simulink model "plant_test"  (R2018a)
settings: Solver=VariableStepAuto  StartTime=0.0  StopTime=10.0  RelTol=1e-3
settings Model: Creator=Rafael  LastModifiedBy=Rafael

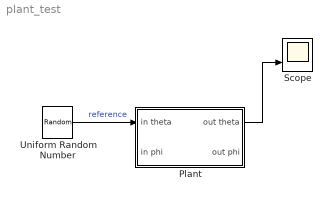
== system plant_test ==
  Plant : Subsystem
  Scope : Scope  NumInputPorts=2
  Uniform Random Number : UniformRandomNumber  Minimum=-1e+6  Maximum=1e+6  SampleTime=1e-6
  wires:
  Uniform Random Number/1 -> Plant/1(in theta)  "reference"
  Plant/1(out theta) -> Scope/2

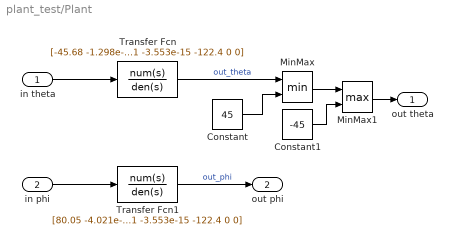
== system plant_test/Plant ==
  in theta : Inport
  in phi : Inport  Port=2
  Constant : Constant  Value=45
  Constant1 : Constant  Value=-45
  MinMax : MinMax  Inputs=2
  MinMax1 : MinMax  Function=max  Inputs=2
  Transfer Fcn : TransferFcn  Numerator=[-45.68 -1.298e-11 7.179e-13]  Denominator=[1 -3.553e-15 -122.4 0 0]
  Transfer Fcn1 : TransferFcn  Numerator=[80.05 -4.021e-12 61140]  Denominator=[1 -3.553e-15 -122.4 0 0]
  out theta : Outport
  out phi : Outport  Port=2
  wires:
  in phi/1 -> Transfer Fcn1/1
  in theta/1 -> Transfer Fcn/1
  Transfer Fcn1/1 -> out phi/1  "out_phi"
  MinMax/1 -> MinMax1/1
  Constant/1 -> MinMax/2
  Constant1/1 -> MinMax1/2
  MinMax1/1 -> out theta/1
  Transfer Fcn/1 -> MinMax/1  "out_theta"
